simulink model "Beobachter"  (R2019a)
settings: Solver=VariableStepAuto  StartTime=0.0  StopTime=10.0  RelTol=1e-3
values from neighbouring files (symbols this model uses):
  A = [0 1 0 0;m*g*l(M+m)/d 0 0 m*l*b/d;0 0 0 1;-g*m^2*l^2/d 0 0 -b*(I+m*l^2)/d]    [inv_pend.m]
  B = [0;-m*l/d;0;(I+m*l^2)/d]    [inv_pend.m]
  C = [0 0 1 0;1 0 0 0]    [inv_pend.m]
  K = acker(A,B,5*[-1 -0.5 -0.4 -0.3])    [inv_pend.m]
  L = place(A',C',[-30 -31 -32 -33])'    [inv_pend.m]
  V = 1/dcgain(ss(A-B*K,B,Cn,Dn))    [inv_pend.m]
settings Model: Creator=Naveen  LastModifiedBy=Naveen

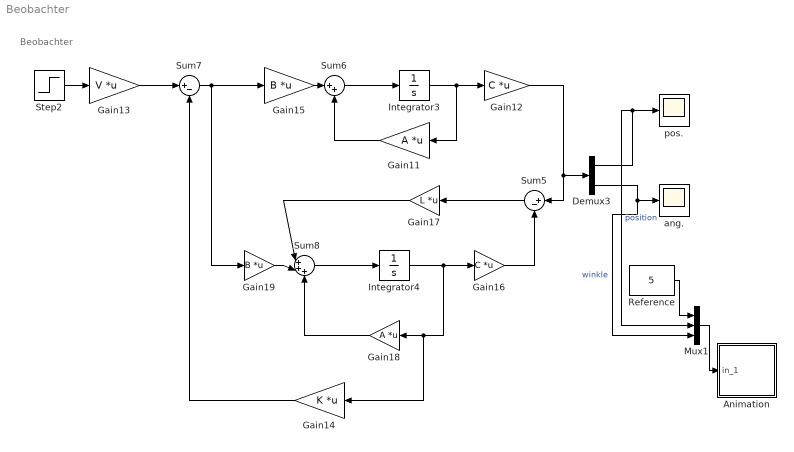
== system Beobachter ==
  note: Beobachter
  Animation : Subsystem  mask(Pendulum plot){RefBlock=Reference}
      mask prompts: RefBlock "DC reference signal block name:"
      mask help: Pendulum plot
      mask Help: Pendulum animation function using Handle graphics.
      mask Display: plot([-10 10],[0 0],[-2 -2 2 2],[0 1 1 0],[0 3],[1 5])
  Demux3 : Demux  Outputs=2
  Gain11 : Gain  Gain=A  Multiplication=Matrix(K*u)
  Gain12 : Gain  Gain=C  Multiplication=Matrix(K*u)
  Gain13 : Gain  Gain=V  Multiplication=Matrix(K*u)
  Gain14 : Gain  Gain=K  Multiplication=Matrix(K*u)
  Gain15 : Gain  Gain=B  Multiplication=Matrix(K*u)
  Gain16 : Gain  Gain=C  Multiplication=Matrix(K*u)
  Gain17 : Gain  Gain=L  Multiplication=Matrix(K*u)
  Gain18 : Gain  Gain=A  Multiplication=Matrix(K*u)
  Gain19 : Gain  Gain=B  Multiplication=Matrix(K*u)
  Integrator3 : Integrator  InitialCondition=[0 0 pi/20 0]
  Integrator4 : Integrator
  Mux1 : Mux  Inputs=3
  Reference : Constant  Value=5
  Step2 : Step  Time=0  After=5  SampleTime=0
  Sum5 : Sum  Inputs=|+-
  Sum6 : Sum  Inputs=|++
  Sum7 : Sum  Inputs=|+-
  Sum8 : Sum  Inputs=|+++
  ang. : Scope
  pos. : Scope
  wires:
  Gain12/1 -> Demux3/1, Sum5/1
  Demux3/2 -> Mux1/3, ang./1  "winkle"
  Gain14/1 -> Sum7/2
  Sum6/1 -> Integrator3/1
  Gain16/1 -> Sum5/2
  Reference/1 -> Mux1/1
  Sum7/1 -> Gain19/1, Gain15/1
  Mux1/1 -> Animation/1(in_1)
  Demux3/1 -> Mux1/2, pos./1  "position"
  Gain11/1 -> Sum6/2
  Step2/1 -> Gain13/1
  Gain13/1 -> Sum7/1
  Gain17/1 -> Sum8/1
  Gain18/1 -> Sum8/3
  Gain19/1 -> Sum8/2
  Sum8/1 -> Integrator4/1
  Integrator4/1 -> Gain14/1, Gain18/1, Gain16/1
  Integrator3/1 -> Gain12/1, Gain11/1
  Gain15/1 -> Sum6/1
  Sum5/1 -> Gain17/1

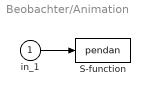
== system Beobachter/Animation ==
  in_1 : Inport
  S-function : S-Function  FunctionName=pendan  Parameters=RefBlock  SFunctionDeploymentMode=off  EnableBusSupport=off
      settings: DeleteFcn=pendan([],[],[],'DeleteBlock');
  wires:
  in_1/1 -> S-function/1
